simulink model "ff_model"  (R2021a)
settings: Solver=VariableStepAuto  StartTime=0.0  StopTime=data.sim.time  RelTol=1e-7  AbsTol=1e-8
values from neighbouring files (symbols this model uses):
  A_i = [A_sc(1); A_sc(2); A_sc(3); A_sc(1); A_sc(2); A_sc(3);            A_sa; A_sa; A_sa; A_sa]'    [data_setup.m]
  n_i = [eye(3), -eye(3), n_sa, -n_sa, n_sa, -n_sa]    [data_setup.m]
  rhoD = ones(1,10)*0.1    [data_setup.m]
  rhoS = [ones(1,6)*0.5, ones(1,4)*0.8]    [data_setup.m]
undefined symbols (not defined in the file or in its folder): data, F107_avg, F107_day, jdate, km, Kp, omega, s
libraries: sharedutil x10, dspmathops x5, aerolibutil x4, dspmtrx3 x3, aerolibcelestial x2, aerolibatmos2 x2, simulink x1, simulink_extras x1
settings Model: Creator=Francesco  LastModifiedBy=Francesco
settings SolverCC: AutoScaleAbsTol=off
settings DataIOCC: SaveFormat=Array  SaveOutput=off  DSMLogging=off  ReturnWorkspaceOutputsName=simout

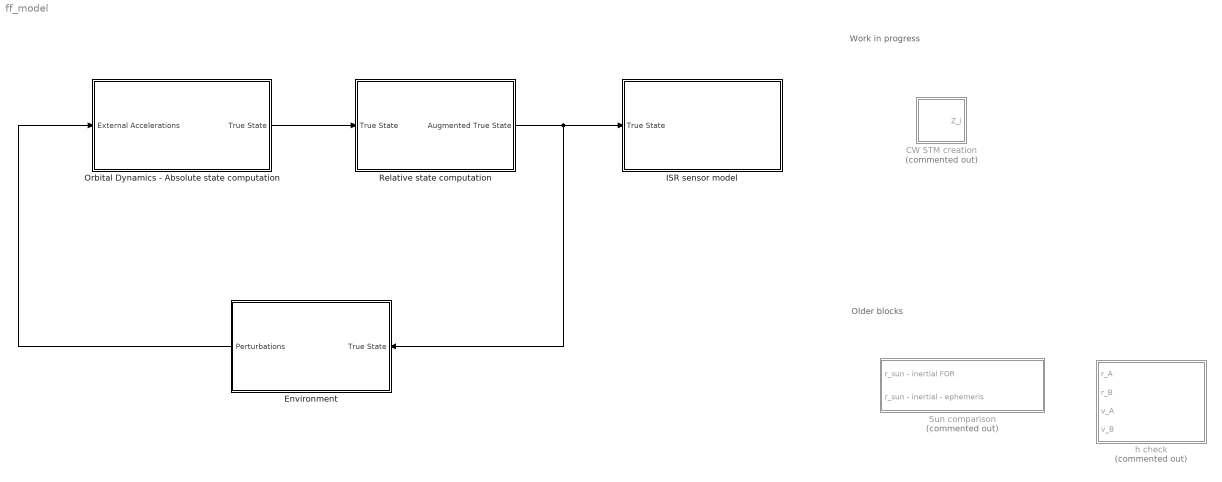
== system ff_model ==
  note: Older blocks
  note: Work in progress
  CW STM creation : Subsystem  Commented=on
  Environment : Subsystem
  ISR sensor model : Subsystem
  "Orbital Dynamics - Absolute state computation " : Subsystem
  Relative state computation : Subsystem
  "Sun comparison " : Subsystem  Commented=on
  h check : Subsystem  Commented=on
  wires:
  Environment/1(Perturbations) -> "Orbital Dynamics - Absolute state computation "/1(External Accelerations)
  "Orbital Dynamics - Absolute state computation "/1(True State) -> Relative state computation/1(True State)
  Relative state computation/1(Augmented True State) -> Environment/1(True State), ISR sensor model/1(True State)

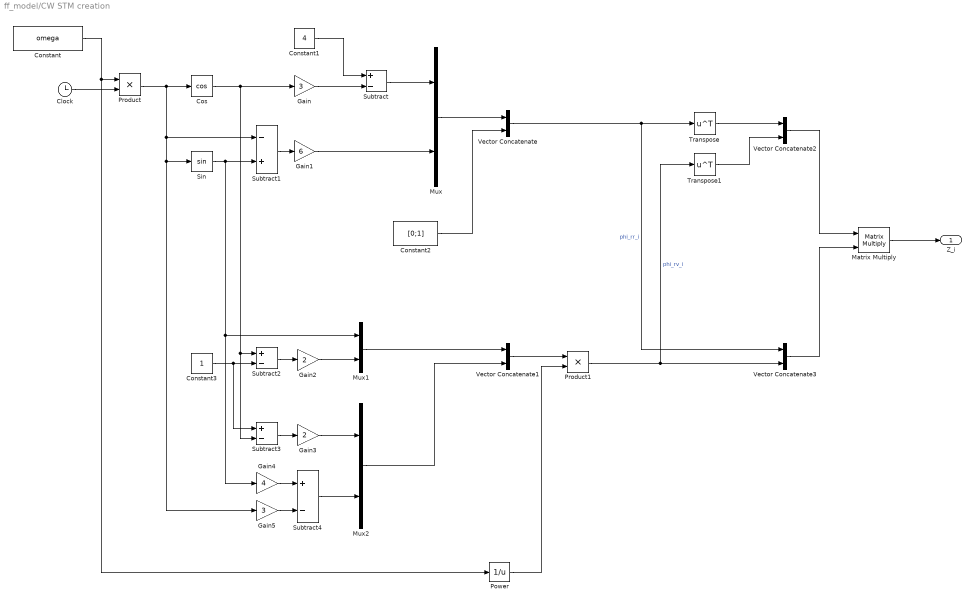
== system ff_model/CW STM creation ==
  Clock : Clock
  Constant : Constant  Value=omega
  Constant1 : Constant  Value=4
  Constant2 : Constant  Value=[0;1]
  Constant3 : Constant
  Cos : Trigonometry  Operator=cos
  Gain : Gain  Gain=3
  Gain1 : Gain  Gain=6
  Gain2 : Gain  Gain=2
  Gain3 : Gain  Gain=2
  Gain4 : Gain  Gain=4
  Gain5 : Gain  Gain=3
  Matrix Multiply : Product  Multiplication=Matrix(*)
  Mux : Mux  Inputs=2
  Mux1 : Mux  Inputs=2
  Mux2 : Mux  Inputs=2
  Power : Math  Operator=reciprocal  SaturateOnIntegerOverflow=on
  Product : Product
  Product1 : Product
  Sin : Trigonometry
  Subtract{,2..4} (4 alike) : Sum  Inputs=+-
  Subtract1 : Sum  Inputs=-+
  Transpose : Math  Operator=transpose  SaturateOnIntegerOverflow=on
  Transpose1 : Math  Operator=transpose  SaturateOnIntegerOverflow=on
  Vector Concatenate : Concatenate  Mode=Multidimensional array  ConcatenateDimension=2
  Vector Concatenate1 : Concatenate  Mode=Multidimensional array  ConcatenateDimension=2
  Vector Concatenate2 : Concatenate  Mode=Multidimensional array
  Vector Concatenate3 : Concatenate  Mode=Multidimensional array  ConcatenateDimension=2
  Z_i : Outport
  wires:
  Product/1 -> Gain5/1, Sin/1, Subtract1/1, Cos/1
  Constant/1 -> Power/1, Product/1
  Gain/1 -> Subtract/2
  Clock/1 -> Product/2
  Subtract/1 -> Mux/1
  Constant2/1 -> Vector Concatenate/2
  Constant1/1 -> Subtract/1
  Cos/1 -> Subtract2/1, Subtract3/2, Gain/1
  Sin/1 -> Gain4/1, Mux1/1, Subtract1/2
  Subtract1/1 -> Gain1/1
  Gain1/1 -> Mux/2
  Mux/1 -> Vector Concatenate/1
  Vector Concatenate/1 -> Vector Concatenate3/1, Transpose/1  "phi_rr_i"
  Constant3/1 -> Subtract3/1, Subtract2/2
  Subtract2/1 -> Gain2/1
  Mux1/1 -> Vector Concatenate1/1
  Gain2/1 -> Mux1/2
  Subtract3/1 -> Gain3/1
  Gain4/1 -> Subtract4/1
  Gain5/1 -> Subtract4/2
  Gain3/1 -> Mux2/1
  Subtract4/1 -> Mux2/2
  Mux2/1 -> Vector Concatenate1/2
  Vector Concatenate1/1 -> Product1/1
  Power/1 -> Product1/2
  Product1/1 -> Transpose1/1, Vector Concatenate3/2  "phi_rv_i"
  Transpose/1 -> Vector Concatenate2/1
  Transpose1/1 -> Vector Concatenate2/2
  Vector Concatenate2/1 -> Matrix Multiply/1
  Vector Concatenate3/1 -> Matrix Multiply/2
  Matrix Multiply/1 -> Z_i/1

== system ff_model/Environment ==
  True State : Inport
  3rd : Scope
  3rd Body : Subsystem
  Drag : Subsystem
  Gain : Gain  Gain=1e-3
  SRP : Subsystem
  Subsystem1 : Subsystem
  Subsystem2 : Subsystem
  Subsystem3 : Subsystem
  Sum : Sum  Inputs=+++
  drag : Scope
  srp : Scope
  Perturbations : Outport
  wires:
  True State/1 -> SRP/1(True State), Drag/1(True State), 3rd Body/1(True State)
  Sum/1 -> Gain/1
  Drag/1(a_drag) -> Subsystem1/1(In1), Sum/3
  3rd Body/1(a_3rd) -> Subsystem2/1(In1), Sum/2
  SRP/1(a_srp) -> Subsystem3/1(In1), Sum/1
  Subsystem3/1(Out1) -> srp/1
  Subsystem2/1(Out1) -> 3rd/1
  Subsystem1/1(Out1) -> drag/1
  Gain/1 -> Perturbations/1

== system ff_model/ISR sensor model ==
  True State : Inport
  Bus Selector : BusSelector  OutputSignals=rel_true_state.posR
  Dot Product : DotProduct  InputSameDT=on  OutDataTypeStr=Inherit: Inherit via internal rule
  Random Number : RandomNumber  Variance=data.sens.sig^2  Seed=354  SampleTime=data.sens.st
  Sqrt : Sqrt  SaturateOnIntegerOverflow=on
  Sum : Sum  Inputs=|++
  To Workspace : ToWorkspace  VariableName=r_meas  SampleTime=-1
      settings: Save2DSignal=2-D array (concatenate along first dimension)
  wires:
  Dot Product/1 -> Sqrt/1
  Sqrt/1 -> Sum/1
  Sum/1 -> To Workspace/1
  Random Number/1 -> Sum/2
  True State/1 -> Bus Selector/1
  Bus Selector/1 -> Dot Product/2, Dot Product/1  "<posR>"

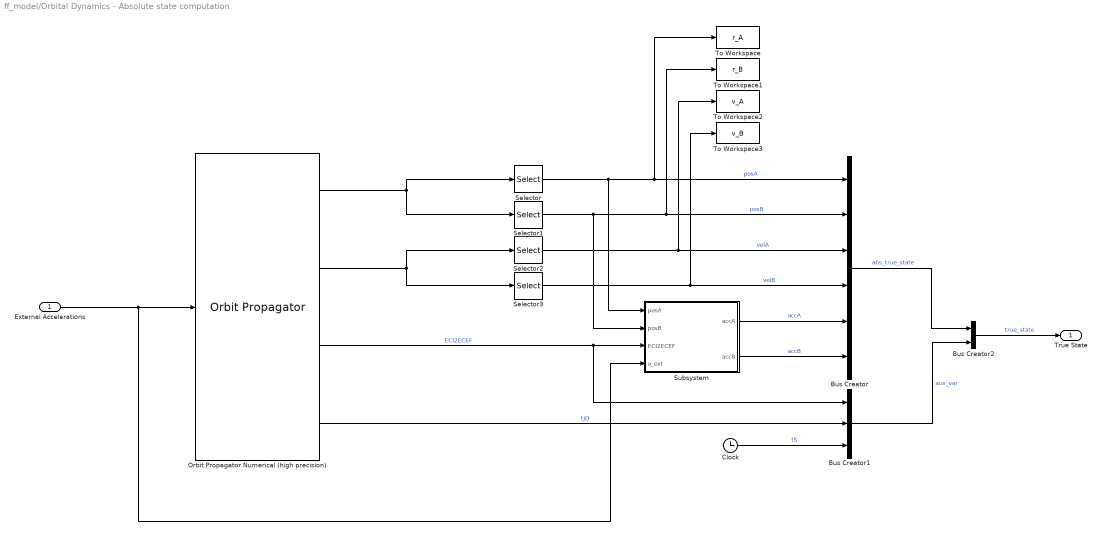
== system ff_model/Orbital Dynamics - Absolute state computation  ==
  External Accelerations : Inport
  Bus Creator : BusCreator  Inputs=6
  Bus Creator1 : BusCreator  Inputs=3
  Bus Creator2 : BusCreator  Inputs=2
  Clock : Clock
  Orbit Propagator Numerical (high precision) : OrbitPropagator  propagator=Numerical (high precision)  accelIn=on  startDate=data.sim.jdate  semiMajorAxis=[data.satA.orbit.a, data.satB.orbit.a]  eccentricity=[data.satA.orbit.e, data.satB.orbit.e]  inclination=[data.satA.orbit.i, data.satB.orbit.i]  raan=[data.satA.orbit.RAAN, data.satB.orbit.RAAN]  argPeriapsis=[data.satA.orbit.om, data.satB.orbit.om]  trueAnomaly=[data.satA.orbit.th, data.satB.orbit.th]  customMu=4.305e13  customJ2=1.0826269e-03  outputTransform=on  units=Metric (km/s)
  Selector : Selector  NumberOfDimensions=2  InputPortWidth=3  IndexOptions=Index vector (dialog),Select all  Indices=1,1  OutputSizes=1,1
  Selector1 : Selector  NumberOfDimensions=2  InputPortWidth=3  IndexOptions=Index vector (dialog),Select all  Indices=2,1  OutputSizes=1,1
  Selector2 : Selector  NumberOfDimensions=2  InputPortWidth=3  IndexOptions=Index vector (dialog),Select all  Indices=1,1  OutputSizes=1,1
  Selector3 : Selector  NumberOfDimensions=2  InputPortWidth=3  IndexOptions=Index vector (dialog),Select all  Indices=2,1  OutputSizes=1,1
  Subsystem : Subsystem
  To Workspace : ToWorkspace  VariableName=r_A  SampleTime=-1
      settings: Save2DSignal=2-D array (concatenate along first dimension)
  To Workspace1 : ToWorkspace  VariableName=r_B  SampleTime=-1
      settings: Save2DSignal=2-D array (concatenate along first dimension)
  To Workspace2 : ToWorkspace  VariableName=v_A  SampleTime=-1
      settings: Save2DSignal=2-D array (concatenate along first dimension)
  To Workspace3 : ToWorkspace  VariableName=v_B  SampleTime=-1
      settings: Save2DSignal=2-D array (concatenate along first dimension)
  True State : Outport
  wires:
  Orbit Propagator Numerical (high precision)/4 -> Bus Creator1/2  "tJD"
  External Accelerations/1 -> Subsystem/4(a_ext), Orbit Propagator Numerical (high precision)/1
  Selector1/1 -> To Workspace1/1, Bus Creator/2, Subsystem/2(posB)  "posB"
  Selector/1 -> To Workspace/1, Bus Creator/1, Subsystem/1(posA)  "posA"
  Orbit Propagator Numerical (high precision)/1 -> Selector/1, Selector1/1
  Orbit Propagator Numerical (high precision)/2 -> Selector2/1, Selector3/1
  Selector2/1 -> To Workspace2/1, Bus Creator/3  "velA"
  Selector3/1 -> To Workspace3/1, Bus Creator/4  "velB"
  Orbit Propagator Numerical (high precision)/3 -> Subsystem/3(ECI2ECEF), Bus Creator1/1  "ECI2ECEF"
  Subsystem/1(accA) -> Bus Creator/5  "accA"
  Subsystem/2(accB) -> Bus Creator/6  "accB"
  Clock/1 -> Bus Creator1/3  "tS"
  Bus Creator1/1 -> Bus Creator2/2  "aux_var"
  Bus Creator/1 -> Bus Creator2/1  "abs_true_state"
  Bus Creator2/1 -> True State/1  "true_state"

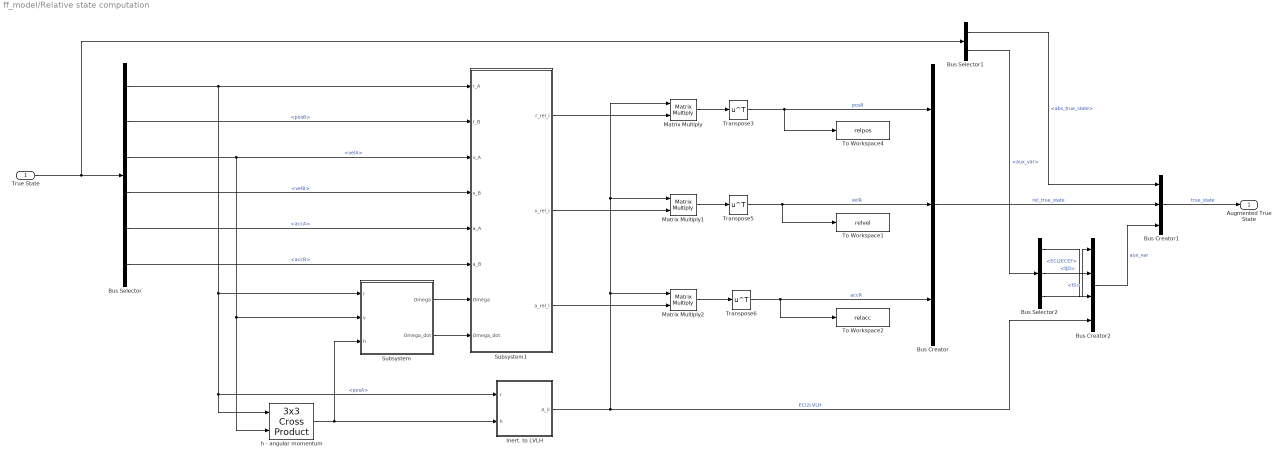
== system ff_model/Relative state computation ==
  True State : Inport
  Bus Creator : BusCreator  Inputs=3
  Bus Creator1 : BusCreator  Inputs=3
  Bus Creator2 : BusCreator  Inputs=4
  Bus Selector : BusSelector  OutputSignals=abs_true_state.posA,abs_true_state.posB,abs_true_state.velA,abs_true_state.velB,abs_true_state.accA,abs_true_state.accB
  Bus Selector1 : BusSelector  OutputSignals=abs_true_state,aux_var
  Bus Selector2 : BusSelector  OutputSignals=ECI2ECEF,tJD,tS
  Inert. to LVLH : Subsystem
  Matrix Multiply : Product  Multiplication=Matrix(*)
  Matrix Multiply1 : Product  Multiplication=Matrix(*)
  Matrix Multiply2 : Product  Multiplication=Matrix(*)
  Subsystem : Subsystem
  Subsystem1 : Subsystem
  To Workspace1 : ToWorkspace  VariableName=relvel  SampleTime=-1
      settings: Save2DSignal=2-D array (concatenate along first dimension)
  To Workspace2 : ToWorkspace  VariableName=relacc  SampleTime=-1
      settings: Save2DSignal=2-D array (concatenate along first dimension)
  To Workspace4 : ToWorkspace  VariableName=relpos  SampleTime=-1
      settings: Save2DSignal=2-D array (concatenate along first dimension)
  Transpose3 : Math  Operator=transpose  SaturateOnIntegerOverflow=on
  Transpose5 : Math  Operator=transpose  SaturateOnIntegerOverflow=on
  Transpose6 : Math  Operator=transpose  SaturateOnIntegerOverflow=on
  h - angular momentum : sharedutil/3x3 Cross Product  aMode=aMode
      settings: SourceProductBaseCode=AE,PW,DR,MT,UV,VE
  Augmented True State : Outport
  wires:
  Inert. to LVLH/1(A_il) -> Bus Creator2/4, Matrix Multiply/1, Matrix Multiply1/1, Matrix Multiply2/1  "ECI2LVLH"
  True State/1 -> Bus Selector1/1, Bus Selector/1
  Bus Selector/4 -> Subsystem1/4(v_B)  "<velB>"
  Bus Selector/5 -> Subsystem1/5(a_A)  "<accA>"
  Bus Selector/2 -> Subsystem1/2(r_B)  "<posB>"
  Bus Selector/1 -> h - angular momentum/1, Inert. to LVLH/1(r), Subsystem/1(r), Subsystem1/1(r_A)  "<posA>"
  Bus Selector/3 -> Subsystem1/3(v_A), h - angular momentum/2, Subsystem/2(v)  "<velA>"
  Bus Selector/6 -> Subsystem1/6(a_B)  "<accB>"
  Subsystem1/3(a_rel_i) -> Matrix Multiply2/2
  Subsystem1/2(v_rel_i) -> Matrix Multiply1/2
  Subsystem1/1(r_rel_i) -> Matrix Multiply/2
  Subsystem/2(Omega_dot) -> Subsystem1/8(Omega_dot)
  Subsystem/1(Omega) -> Subsystem1/7(Omega)
  Matrix Multiply2/1 -> Transpose6/1
  Transpose6/1 -> Bus Creator/3, To Workspace2/1  "accR"
  Transpose3/1 -> To Workspace4/1, Bus Creator/1  "posR"
  Transpose5/1 -> Bus Creator/2, To Workspace1/1  "velR"
  Matrix Multiply1/1 -> Transpose5/1
  Matrix Multiply/1 -> Transpose3/1
  h - angular momentum/1 -> Inert. to LVLH/2(h), Subsystem/3(h)
  Bus Creator/1 -> Bus Creator1/2  "rel_true_state"
  Bus Creator1/1 -> Augmented True State/1  "true_state"
  Bus Selector1/1 -> Bus Creator1/1  "<abs_true_state>"
  Bus Selector1/2 -> Bus Selector2/1  "<aux_var>"
  Bus Selector2/3 -> Bus Creator2/1  "<tS>"
  Bus Selector2/2 -> Bus Creator2/2  "<tJD>"
  Bus Selector2/1 -> Bus Creator2/3  "<ECI2ECEF>"
  Bus Creator2/1 -> Bus Creator1/3  "aux_var"

== system ff_model/Sun comparison  ==
  r_sun - inertial FOR : Inport
  r_sun - inertial - ephemeris : Inport  Port=2
  Acos : Trigonometry  Operator=acos
  Dot Product : DotProduct  InputSameDT=on  OutDataTypeStr=Inherit: Inherit via internal rule
  Radians to Degrees : simulink_extras/Transformations/Radians to Degrees
  Scope : Scope  NumInputPorts=2
  Scope2 : Scope
  wires:
  Acos/1 -> Radians to Degrees/1
  Dot Product/1 -> Acos/1
  r_sun - inertial - ephemeris/1 -> Scope/2, Dot Product/2
  Radians to Degrees/1 -> Scope2/1
  r_sun - inertial FOR/1 -> Scope/1, Dot Product/1

== system ff_model/h check ==
  r_A : Inport
  r_B : Inport  Port=2
  v_A : Inport  Port=3
  v_B : Inport  Port=4
  3x3 Cross Product : sharedutil/3x3 Cross Product  aMode=aMode
      settings: SourceProductBaseCode=AE,PW,DR,MT,UV,VE
  3x3 Cross Product1 : sharedutil/3x3 Cross Product  aMode=aMode
      settings: SourceProductBaseCode=AE,PW,DR,MT,UV,VE
  Scope6 : Scope  Commented=on  NumInputPorts=2
  Subsystem : Subsystem
  Subsystem1 : Subsystem
  wires:
  r_B/1 -> 3x3 Cross Product1/1
  3x3 Cross Product/1 -> Subsystem/1(vec)
  3x3 Cross Product1/1 -> Subsystem1/1(vec)
  Subsystem1/1(norm) -> Scope6/2
  Subsystem/1(norm) -> Scope6/1
  v_B/1 -> 3x3 Cross Product1/2
  v_A/1 -> 3x3 Cross Product/2
  r_A/1 -> 3x3 Cross Product/1

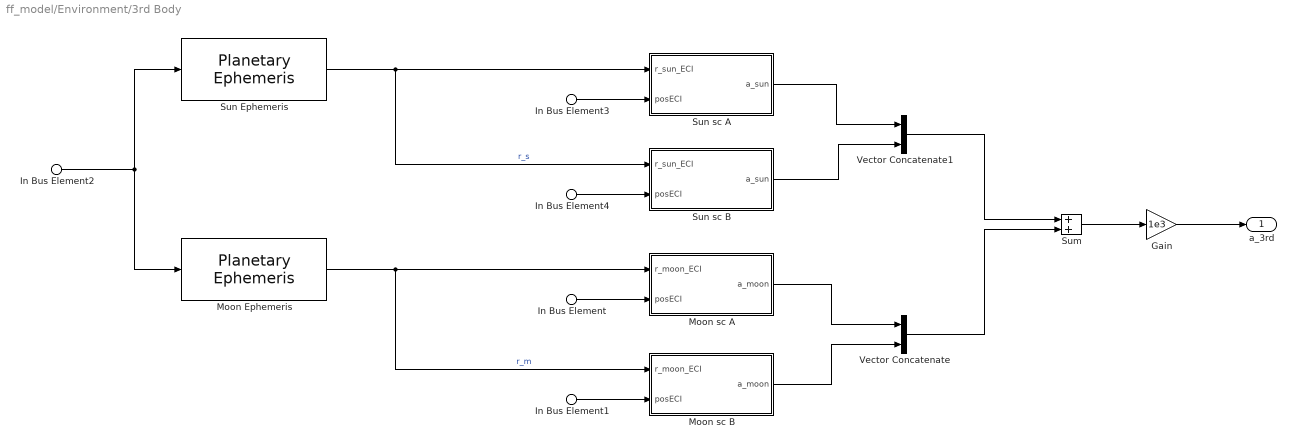
== system ff_model/Environment/3rd Body ==
  In Bus Element : Inport  PortName=True State  Element=abs_true_state.posA
  In Bus Element3 : Inport  PortName=True State  Element=abs_true_state.posA
  In Bus Element1 : Inport  PortName=True State  Element=abs_true_state.posB
  In Bus Element4 : Inport  PortName=True State  Element=abs_true_state.posB
  In Bus Element2 : Inport  PortName=True State  Element=aux_var.tJD
  Gain : Gain  Gain=1e3
  Moon Ephemeris : aerolibcelestial/Planetary Ephemeris  kmflag=km,km/s  epochflag=Julian date  de=DE405  nCenter=Earth  nTarget=Moon  errorflag=Error  velflag=off
      settings: SourceProductBaseCode=AE
  "Moon sc A " : Subsystem
  Moon sc B : Subsystem
  Sum : Sum
  Sun Ephemeris : aerolibcelestial/Planetary Ephemeris  kmflag=km,km/s  epochflag=Julian date  de=DE405  nCenter=Earth  nTarget=Sun  errorflag=Error  velflag=off
      settings: SourceProductBaseCode=AE
  Sun sc A : Subsystem
  Sun sc B : Subsystem
  Vector Concatenate : Concatenate  Mode=Multidimensional array
  Vector Concatenate1 : Concatenate  Mode=Multidimensional array
  a_3rd : Outport
  wires:
  In Bus Element2/1 -> Moon Ephemeris/1, Sun Ephemeris/1
  Moon Ephemeris/1 -> Moon sc B/1(r_moon_ECI), "Moon sc A "/1(r_moon_ECI)  "r_m"
  In Bus Element/1 -> "Moon sc A "/2(posECI)
  In Bus Element1/1 -> Moon sc B/2(posECI)
  Vector Concatenate/1 -> Sum/2
  "Moon sc A "/1(a_moon) -> Vector Concatenate/1
  Moon sc B/1(a_moon) -> Vector Concatenate/2
  Sun sc B/1(a_sun) -> Vector Concatenate1/2
  In Bus Element3/1 -> Sun sc A/2(posECI)
  Sun sc A/1(a_sun) -> Vector Concatenate1/1
  Sun Ephemeris/1 -> Sun sc B/1(r_sun_ECI), Sun sc A/1(r_sun_ECI)  "r_s"
  Vector Concatenate1/1 -> Sum/1
  In Bus Element4/1 -> Sun sc B/2(posECI)
  Sum/1 -> Gain/1
  Gain/1 -> a_3rd/1

== system ff_model/Environment/Drag ==
  In Bus Element : Inport  PortName=True State  Element=abs_true_state.posA
  In Bus Element1 : Inport  PortName=True State  Element=abs_true_state.posB
  In Bus Element2 : Inport  PortName=True State  Element=abs_true_state.velA
  In Bus Element3 : Inport  PortName=True State  Element=abs_true_state.velB
  In Bus Element4 : Inport  PortName=True State  Element=aux_var.ECI2ECEF
  Density sc A : Subsystem
  Density sc B : Subsystem
  Drag sc A : Subsystem
  Drag sc B : Subsystem
  Vector Concatenate : Concatenate  Mode=Multidimensional array
  check rho Jacchia : Subsystem  Commented=on
  rho comp : Scope  Commented=on  NumInputPorts=2
  a_drag : Outport
  wires:
  In Bus Element1/1 -> Drag sc B/3(posECI), Density sc B/2(posECI)
  In Bus Element4/1 -> Density sc A/1(ECI2ECEF), Density sc B/1(ECI2ECEF)
  In Bus Element/1 -> Drag sc A/3(posECI), check rho Jacchia/2(vec), Density sc A/2(posECI)
  Drag sc A/1(a_drag) -> Vector Concatenate/1
  Drag sc B/1(a_drag) -> Vector Concatenate/2
  Vector Concatenate/1 -> a_drag/1
  Density sc B/1(rho) -> Drag sc B/2(rho)
  Density sc A/1(rho) -> check rho Jacchia/1(In1), Drag sc A/2(rho)
  In Bus Element2/1 -> Drag sc A/1(velECI)
  In Bus Element3/1 -> Drag sc B/1(velECI)
  check rho Jacchia/1(Out1) -> rho comp/1
  check rho Jacchia/2(Out2) -> rho comp/2

== system ff_model/Environment/SRP ==
  True State : Inport
  Bus Selector : BusSelector  OutputSignals=aux_var.ECI2LVLH,abs_true_state.posA
  SRP : Subsystem
  Sun Position : Subsystem
  Transpose : Math  Operator=transpose  SaturateOnIntegerOverflow=on
  Vector Concatenate : Concatenate  Mode=Multidimensional array
  a_srp : Outport
  wires:
  Vector Concatenate/1 -> a_srp/1
  True State/1 -> Bus Selector/1
  Sun Position/1(r_sun - inertial FOR) -> SRP/2(r_sun - inertial FOR)
  Transpose/1 -> Vector Concatenate/2, Vector Concatenate/1
  SRP/1(a_SRP_Inert) -> Transpose/1
  Sun Position/2(Shadow) -> SRP/3(Shadow)
  Bus Selector/2 -> Sun Position/1(r_sc - inert FOR)  "<posA>"
  Bus Selector/1 -> SRP/1(A_il)  "<ECI2LVLH>"

== system ff_model/Environment/Subsystem1 ==
  In1 : Inport
  Extract Diagonal : dspmtrx3/Extract Diagonal
      settings: SourceProductBaseCode=DS
  Matrix Multiply : Product  Multiplication=Matrix(*)
  Sqrt : Sqrt  SaturateOnIntegerOverflow=on
  Transpose : Math  Operator=transpose  SaturateOnIntegerOverflow=on
  Out1 : Outport
  wires:
  In1/1 -> Transpose/1, Matrix Multiply/1
  Transpose/1 -> Matrix Multiply/2
  Matrix Multiply/1 -> Extract Diagonal/1
  Extract Diagonal/1 -> Sqrt/1
  Sqrt/1 -> Out1/1

== system ff_model/Environment/Subsystem2 ==
  In1 : Inport
  Extract Diagonal : dspmtrx3/Extract Diagonal
      settings: SourceProductBaseCode=DS
  Matrix Multiply : Product  Multiplication=Matrix(*)
  Sqrt : Sqrt  SaturateOnIntegerOverflow=on
  Transpose : Math  Operator=transpose  SaturateOnIntegerOverflow=on
  Out1 : Outport
  wires:
  In1/1 -> Transpose/1, Matrix Multiply/1
  Transpose/1 -> Matrix Multiply/2
  Matrix Multiply/1 -> Extract Diagonal/1
  Extract Diagonal/1 -> Sqrt/1
  Sqrt/1 -> Out1/1

== system ff_model/Environment/Subsystem3 ==
  In1 : Inport
  Extract Diagonal : dspmtrx3/Extract Diagonal
      settings: SourceProductBaseCode=DS
  Matrix Multiply : Product  Multiplication=Matrix(*)
  Sqrt : Sqrt  SaturateOnIntegerOverflow=on
  Transpose : Math  Operator=transpose  SaturateOnIntegerOverflow=on
  Out1 : Outport
  wires:
  In1/1 -> Transpose/1, Matrix Multiply/1
  Transpose/1 -> Matrix Multiply/2
  Matrix Multiply/1 -> Extract Diagonal/1
  Extract Diagonal/1 -> Sqrt/1
  Sqrt/1 -> Out1/1

== system ff_model/Orbital Dynamics - Absolute state computation /Subsystem ==
  posA : Inport
  posB : Inport  Port=2
  ECI2ECEF : Inport  Port=3
  a_ext : Inport  Port=4
  Gain : Gain  Gain=1e3
  Quaternion Rotation : aerolibutil/Quaternion Rotation
  Quaternion Rotation1 : aerolibutil/Quaternion Rotation
  Selector : Selector  NumberOfDimensions=2  InputPortWidth=3  IndexOptions=Index vector (dialog),Select all  Indices=1,1  OutputSizes=1,1
  Selector1 : Selector  NumberOfDimensions=2  InputPortWidth=3  IndexOptions=Index vector (dialog),Select all  Indices=2,1  OutputSizes=1,1
  Spherical Harmonic Gravity Model : SHGravity
  Sum : Sum  Inputs=|++
  Transpose : Math  Operator=transpose  SaturateOnIntegerOverflow=on
  Vector Concatenate : Concatenate  Mode=Multidimensional array  ConcatenateDimension=2
  accA : Outport
  accB : Outport  Port=2
  wires:
  Quaternion Rotation/1 -> Vector Concatenate/1
  Spherical Harmonic Gravity Model/1 -> Sum/1
  ECI2ECEF/1 -> Quaternion Rotation1/1, Quaternion Rotation/1
  posA/1 -> Quaternion Rotation/2
  posB/1 -> Quaternion Rotation1/2
  Vector Concatenate/1 -> Transpose/1
  Quaternion Rotation1/1 -> Vector Concatenate/2
  Transpose/1 -> Gain/1
  a_ext/1 -> Sum/2
  Sum/1 -> Selector1/1, Selector/1
  Selector/1 -> accA/1  "accA"
  Selector1/1 -> accB/1  "accB"
  Gain/1 -> Spherical Harmonic Gravity Model/1

== system ff_model/Relative state computation/Inert. to LVLH ==
  r : Inport
  h : Inport  Port=2
  3x3 Cross Product1 : sharedutil/3x3 Cross Product  aMode=aMode
      settings: SourceProductBaseCode=AE,PW,DR,MT,UV,VE
  Normalization : dspmathops/Normalization  NormType=2-norm  Bias=1e-10  NormOver=Each row  Dimension=1  roundingMode=Floor  overflowMode=off  accumDataTypeStr=Inherit: Same as product output  accumLastDataTypeStr=Inherit: Same as product output  outputDataTypeStr=Inherit: Same as product output  outputMin=[]  outputMax=[]  outputLastDataTypeStr=Inherit: Same as product output
  Normalization2 : dspmathops/Normalization  NormType=2-norm  Bias=1e-10  NormOver=Each row  Dimension=1  roundingMode=Floor  overflowMode=off  accumDataTypeStr=Inherit: Same as product output  accumLastDataTypeStr=Inherit: Same as product output  outputDataTypeStr=Inherit: Same as product output  outputMin=[]  outputMax=[]  outputLastDataTypeStr=Inherit: Same as product output
  Transpose : Math  Operator=transpose  SaturateOnIntegerOverflow=on
  Transpose1 : Math  Operator=transpose  SaturateOnIntegerOverflow=on
  Vector Concatenate : Concatenate  NumInputs=3  Mode=Multidimensional array
  A_il : Outport
  wires:
  Normalization2/1 -> 3x3 Cross Product1/1, Transpose/1
  h/1 -> Normalization2/1
  3x3 Cross Product1/1 -> Transpose1/1
  Normalization/1 -> Vector Concatenate/1, 3x3 Cross Product1/2  "x_hat"
  Vector Concatenate/1 -> A_il/1
  r/1 -> Normalization/1
  Transpose1/1 -> Vector Concatenate/2  "y_hat"
  Transpose/1 -> Vector Concatenate/3  "z_hat"

== system ff_model/Relative state computation/Subsystem ==
  r : Inport
  v : Inport  Port=2
  h : Inport  Port=3
  Divide : Product  Inputs=*/
  Divide1 : Product  Inputs=*/
  Dot Product : DotProduct  InputSameDT=on  OutDataTypeStr=Inherit: Inherit via internal rule
  Dot Product1 : DotProduct  InputSameDT=on  OutDataTypeStr=Inherit: Inherit via internal rule
  Gain2 : Gain  Gain=-2
  Product : Product
  Omega : Outport
  Omega_dot : Outport  Port=2
  wires:
  Product/1 -> Omega_dot/1  "Omega_dot"
  Divide1/1 -> Product/2  "Omega"
  Dot Product1/1 -> Gain2/1
  r/1 -> Dot Product/2, Dot Product1/2, Dot Product/1
  h/1 -> Divide/1
  v/1 -> Dot Product1/1
  Gain2/1 -> Divide1/1
  Divide/1 -> Product/1, Omega/1  "Omega"
  Dot Product/1 -> Divide1/2, Divide/2

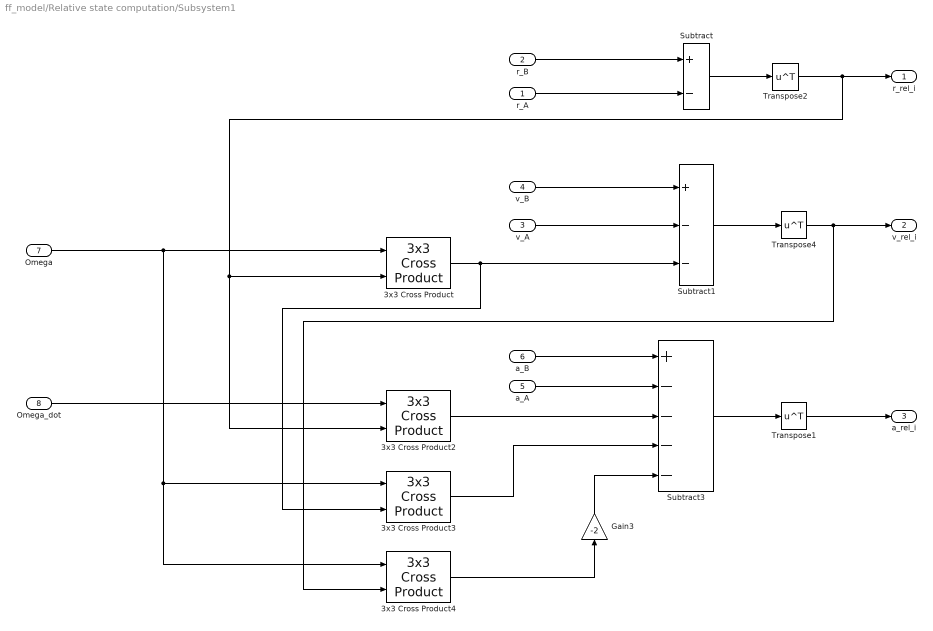
== system ff_model/Relative state computation/Subsystem1 ==
  r_A : Inport
  r_B : Inport  Port=2
  v_A : Inport  Port=3
  v_B : Inport  Port=4
  a_A : Inport  Port=5
  a_B : Inport  Port=6
  Omega : Inport  Port=7
  Omega_dot : Inport  Port=8
  3x3 Cross Product{,2..4} (4 alike) : sharedutil/3x3 Cross Product  aMode=aMode
      settings: SourceProductBaseCode=AE,PW,DR,MT,UV,VE
  Gain3 : Gain  Gain=-2
  Subtract : Sum  Inputs=+-
  Subtract1 : Sum  Inputs=+--
  Subtract3 : Sum  Inputs=+----
  Transpose1 : Math  Operator=transpose  SaturateOnIntegerOverflow=on
  Transpose2 : Math  Operator=transpose  SaturateOnIntegerOverflow=on
  Transpose4 : Math  Operator=transpose  SaturateOnIntegerOverflow=on
  r_rel_i : Outport
  v_rel_i : Outport  Port=2
  a_rel_i : Outport  Port=3
  wires:
  Omega/1 -> 3x3 Cross Product4/1, 3x3 Cross Product3/1, 3x3 Cross Product/1
  Subtract1/1 -> Transpose4/1
  Subtract/1 -> Transpose2/1
  Transpose2/1 -> 3x3 Cross Product/2, 3x3 Cross Product2/2, r_rel_i/1
  3x3 Cross Product/1 -> Subtract1/3, 3x3 Cross Product3/2
  Transpose4/1 -> 3x3 Cross Product4/2, v_rel_i/1
  r_B/1 -> Subtract/1
  Gain3/1 -> Subtract3/5
  3x3 Cross Product2/1 -> Subtract3/3
  3x3 Cross Product4/1 -> Gain3/1
  3x3 Cross Product3/1 -> Subtract3/4
  r_A/1 -> Subtract/2
  v_A/1 -> Subtract1/2
  Omega_dot/1 -> 3x3 Cross Product2/1
  a_A/1 -> Subtract3/2
  a_B/1 -> Subtract3/1
  v_B/1 -> Subtract1/1
  Subtract3/1 -> Transpose1/1
  Transpose1/1 -> a_rel_i/1

== system ff_model/h check/Subsystem ==
  vec : Inport
  Dot Product : DotProduct  InputSameDT=on  OutDataTypeStr=Inherit: Inherit via internal rule
  Sqrt : Sqrt  SaturateOnIntegerOverflow=on
  norm : Outport
  wires:
  Dot Product/1 -> Sqrt/1
  vec/1 -> Dot Product/2, Dot Product/1
  Sqrt/1 -> norm/1

== system ff_model/h check/Subsystem1 ==
  vec : Inport
  Dot Product : DotProduct  InputSameDT=on  OutDataTypeStr=Inherit: Inherit via internal rule
  Sqrt : Sqrt  SaturateOnIntegerOverflow=on
  norm : Outport
  wires:
  Dot Product/1 -> Sqrt/1
  vec/1 -> Dot Product/2, Dot Product/1
  Sqrt/1 -> norm/1

== system ff_model/Environment/3rd Body/Moon sc A  ==
  r_moon_ECI : Inport
  posECI : Inport  Port=2
  Constant : Constant  Value=data.env.mi_moon
  Constant1 : Constant  Value=3
  Constant2 : Constant  Value=3
  Divide : Product  Inputs=*/
  Divide1 : Product  Inputs=*/
  Power : Math  Operator=pow  SaturateOnIntegerOverflow=on
  Power1 : Math  Operator=pow  SaturateOnIntegerOverflow=on
  Product : Product
  Subsystem : Subsystem
  Subsystem1 : Subsystem
  Subtract : Sum  Inputs=+-
  Subtract1 : Sum  Inputs=+-
  a_moon : Outport
  wires:
  Divide1/1 -> Subtract1/2
  r_moon_ECI/1 -> Subtract/1, Subsystem1/1(vec), Divide1/1
  Constant1/1 -> Power/2
  Subtract/1 -> Subsystem/1(vec), Divide/1  "r_sc_m"
  Power/1 -> Divide/2
  Divide/1 -> Subtract1/1
  Power1/1 -> Divide1/2
  Constant2/1 -> Power1/2
  Subsystem1/1(norm) -> Power1/1
  Constant/1 -> Product/1
  Subtract1/1 -> Product/2
  Subsystem/1(norm) -> Power/1
  posECI/1 -> Subtract/2
  Product/1 -> a_moon/1

== system ff_model/Environment/3rd Body/Moon sc B ==
  r_moon_ECI : Inport
  posECI : Inport  Port=2
  Constant : Constant  Value=data.env.mi_moon
  Constant1 : Constant  Value=3
  Constant2 : Constant  Value=3
  Divide : Product  Inputs=*/
  Divide1 : Product  Inputs=*/
  Power : Math  Operator=pow  SaturateOnIntegerOverflow=on
  Power1 : Math  Operator=pow  SaturateOnIntegerOverflow=on
  Product : Product
  Subsystem : Subsystem
  Subsystem1 : Subsystem
  Subtract : Sum  Inputs=+-
  Subtract1 : Sum  Inputs=+-
  a_moon : Outport
  wires:
  Divide1/1 -> Subtract1/2
  r_moon_ECI/1 -> Subtract/1, Subsystem1/1(vec), Divide1/1
  Constant1/1 -> Power/2
  Subtract/1 -> Subsystem/1(vec), Divide/1  "r_sc_m"
  Power/1 -> Divide/2
  Divide/1 -> Subtract1/1
  Power1/1 -> Divide1/2
  Constant2/1 -> Power1/2
  Subsystem1/1(norm) -> Power1/1
  Constant/1 -> Product/1
  Subtract1/1 -> Product/2
  Subsystem/1(norm) -> Power/1
  posECI/1 -> Subtract/2
  Product/1 -> a_moon/1

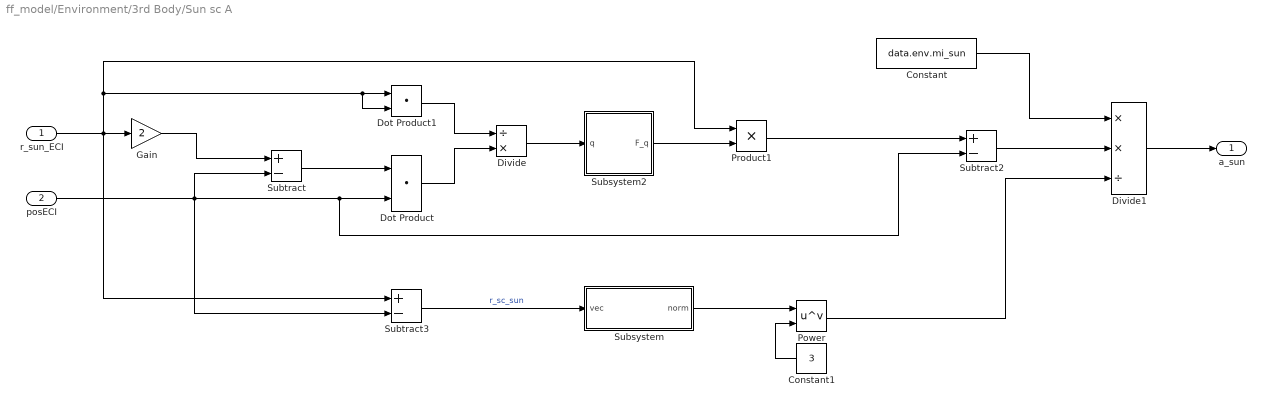
== system ff_model/Environment/3rd Body/Sun sc A ==
  r_sun_ECI : Inport
  posECI : Inport  Port=2
  Constant : Constant  Value=data.env.mi_sun
  Constant1 : Constant  Value=3
  Divide : Product  Inputs=/*
  Divide1 : Product  Inputs=**/
  Dot Product : DotProduct  InputSameDT=on  OutDataTypeStr=Inherit: Inherit via internal rule
  Dot Product1 : DotProduct  InputSameDT=on  OutDataTypeStr=Inherit: Inherit via internal rule
  Gain : Gain  Gain=2
  Power : Math  Operator=pow  SaturateOnIntegerOverflow=on
  Product1 : Product
  Subsystem : Subsystem
  Subsystem2 : Subsystem
  Subtract : Sum  Inputs=+-
  Subtract2 : Sum  Inputs=+-
  Subtract3 : Sum  Inputs=+-
  a_sun : Outport
  wires:
  r_sun_ECI/1 -> Product1/1, Dot Product1/2, Dot Product1/1, Subtract3/1, Gain/1
  Gain/1 -> Subtract/1
  Subtract/1 -> Dot Product/1
  Dot Product1/1 -> Divide/1
  Dot Product/1 -> Divide/2
  Divide/1 -> Subsystem2/1(q)
  Subsystem2/1(F_q) -> Product1/2
  Product1/1 -> Subtract2/1
  posECI/1 -> Subtract3/2, Subtract2/2, Dot Product/2, Subtract/2
  Power/1 -> Divide1/3
  Constant1/1 -> Power/2
  Subtract3/1 -> Subsystem/1(vec)  "r_sc_sun"
  Subsystem/1(norm) -> Power/1
  Constant/1 -> Divide1/1
  Subtract2/1 -> Divide1/2
  Divide1/1 -> a_sun/1

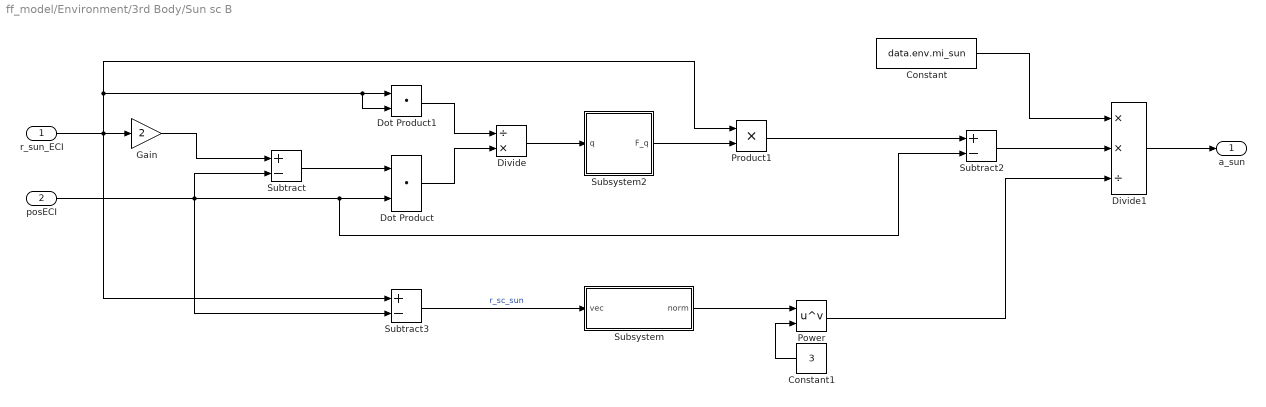
== system ff_model/Environment/3rd Body/Sun sc B ==
  r_sun_ECI : Inport
  posECI : Inport  Port=2
  Constant : Constant  Value=data.env.mi_sun
  Constant1 : Constant  Value=3
  Divide : Product  Inputs=/*
  Divide1 : Product  Inputs=**/
  Dot Product : DotProduct  InputSameDT=on  OutDataTypeStr=Inherit: Inherit via internal rule
  Dot Product1 : DotProduct  InputSameDT=on  OutDataTypeStr=Inherit: Inherit via internal rule
  Gain : Gain  Gain=2
  Power : Math  Operator=pow  SaturateOnIntegerOverflow=on
  Product1 : Product
  Subsystem : Subsystem
  Subsystem2 : Subsystem
  Subtract : Sum  Inputs=+-
  Subtract2 : Sum  Inputs=+-
  Subtract3 : Sum  Inputs=+-
  a_sun : Outport
  wires:
  r_sun_ECI/1 -> Product1/1, Dot Product1/2, Dot Product1/1, Subtract3/1, Gain/1
  Gain/1 -> Subtract/1
  Subtract/1 -> Dot Product/1
  Dot Product1/1 -> Divide/1
  Dot Product/1 -> Divide/2
  Divide/1 -> Subsystem2/1(q)
  Subsystem2/1(F_q) -> Product1/2
  Product1/1 -> Subtract2/1
  posECI/1 -> Subtract3/2, Subtract2/2, Dot Product/2, Subtract/2
  Power/1 -> Divide1/3
  Constant1/1 -> Power/2
  Subtract3/1 -> Subsystem/1(vec)  "r_sc_sun"
  Subsystem/1(norm) -> Power/1
  Constant/1 -> Divide1/1
  Subtract2/1 -> Divide1/2
  Divide1/1 -> a_sun/1

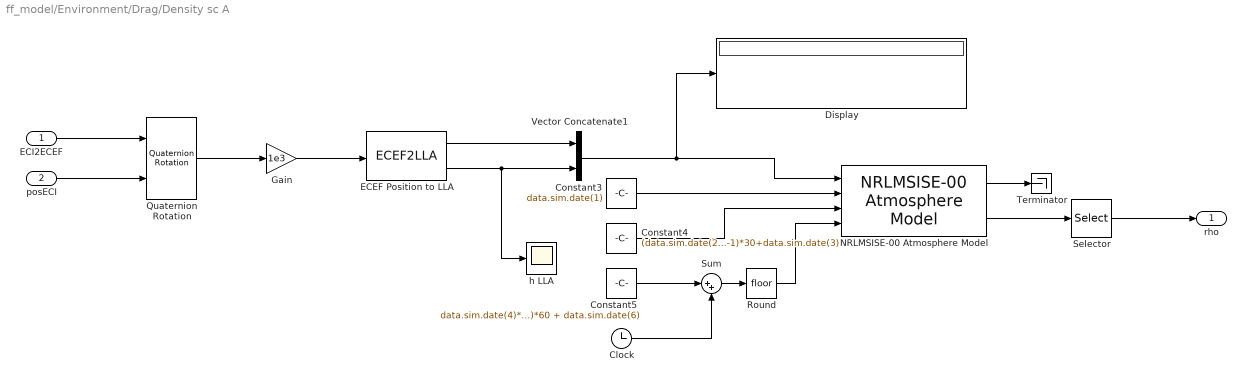
== system ff_model/Environment/Drag/Density sc A ==
  ECI2ECEF : Inport
  posECI : Inport  Port=2
  Clock : Clock
  Constant3 : Constant  Value=data.sim.date(1)
  Constant4 : Constant  Value=(data.sim.date(2)-1)*30+data.sim.date(3)
  Constant5 : Constant  Value=data.sim.date(4)*60*60 + data.sim.date(5)*60 + data.sim.date(6)
  Display : Display
  ECEF Position to LLA : ECEF2LLA
  Gain : Gain  Gain=1e3
  NRLMSISE-00 Atmosphere Model : aerolibatmos2/NRLMSISE-00 Atmosphere Model  units=Metric (MKS)  lst_input=off  flux_ap_input=off  flags_input=Internal  flags=ones(1,23)  oxygen_in=on  action=Warning
      settings: SourceProductBaseCode=AE
  Quaternion Rotation : aerolibutil/Quaternion Rotation
  Round : Rounding
  Selector : Selector  InputPortWidth=9  IndexOptions=Index vector (dialog)  Indices=6  OutputSizes=1
  Sum : Sum  Inputs=|++
  Terminator : Terminator
  Vector Concatenate1 : Concatenate
  h LLA : Scope
  rho : Outport
  wires:
  Constant4/1 -> NRLMSISE-00 Atmosphere Model/3
  Gain/1 -> ECEF Position to LLA/1
  Vector Concatenate1/1 -> Display/1, NRLMSISE-00 Atmosphere Model/1
  Clock/1 -> Sum/2
  NRLMSISE-00 Atmosphere Model/1 -> Terminator/1
  NRLMSISE-00 Atmosphere Model/2 -> Selector/1
  ECEF Position to LLA/1 -> Vector Concatenate1/1
  Constant3/1 -> NRLMSISE-00 Atmosphere Model/2
  Quaternion Rotation/1 -> Gain/1
  Constant5/1 -> Sum/1
  Sum/1 -> Round/1
  ECEF Position to LLA/2 -> h LLA/1, Vector Concatenate1/2
  Selector/1 -> rho/1
  Round/1 -> NRLMSISE-00 Atmosphere Model/4
  posECI/1 -> Quaternion Rotation/2
  ECI2ECEF/1 -> Quaternion Rotation/1

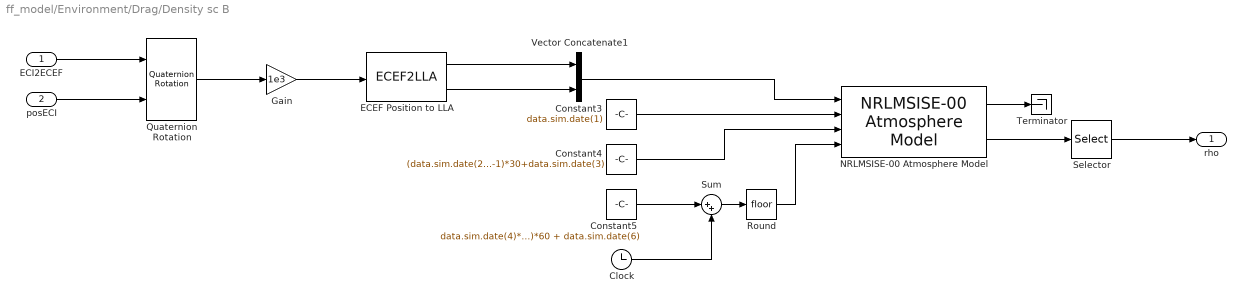
== system ff_model/Environment/Drag/Density sc B ==
  ECI2ECEF : Inport
  posECI : Inport  Port=2
  Clock : Clock
  Constant3 : Constant  Value=data.sim.date(1)
  Constant4 : Constant  Value=(data.sim.date(2)-1)*30+data.sim.date(3)
  Constant5 : Constant  Value=data.sim.date(4)*60*60 + data.sim.date(5)*60 + data.sim.date(6)
  ECEF Position to LLA : ECEF2LLA
  Gain : Gain  Gain=1e3
  NRLMSISE-00 Atmosphere Model : aerolibatmos2/NRLMSISE-00 Atmosphere Model  units=Metric (MKS)  lst_input=off  flux_ap_input=off  flags_input=Internal  flags=ones(1,23)  oxygen_in=on  action=Warning
      settings: SourceProductBaseCode=AE
  Quaternion Rotation : aerolibutil/Quaternion Rotation
  Round : Rounding
  Selector : Selector  InputPortWidth=9  IndexOptions=Index vector (dialog)  Indices=6  OutputSizes=1
  Sum : Sum  Inputs=|++
  Terminator : Terminator
  Vector Concatenate1 : Concatenate
  rho : Outport
  wires:
  Constant4/1 -> NRLMSISE-00 Atmosphere Model/3
  Gain/1 -> ECEF Position to LLA/1
  Vector Concatenate1/1 -> NRLMSISE-00 Atmosphere Model/1
  Clock/1 -> Sum/2
  NRLMSISE-00 Atmosphere Model/1 -> Terminator/1
  NRLMSISE-00 Atmosphere Model/2 -> Selector/1
  ECEF Position to LLA/1 -> Vector Concatenate1/1
  Constant3/1 -> NRLMSISE-00 Atmosphere Model/2
  Quaternion Rotation/1 -> Gain/1
  Constant5/1 -> Sum/1
  Sum/1 -> Round/1
  ECEF Position to LLA/2 -> Vector Concatenate1/2
  Selector/1 -> rho/1
  Round/1 -> NRLMSISE-00 Atmosphere Model/4
  posECI/1 -> Quaternion Rotation/2
  ECI2ECEF/1 -> Quaternion Rotation/1

== system ff_model/Environment/Drag/Drag sc A ==
  velECI : Inport
  rho : Inport  Port=2
  posECI : Inport  Port=3
  3x3 Cross Product : sharedutil/3x3 Cross Product  aMode=aMode
      settings: SourceProductBaseCode=AE,PW,DR,MT,UV,VE
  Constant : Constant  Value=[0 0 data.env.w_e]
  Constant1 : Constant  Value=-0.5
  Constant2 : Constant  Value=data.satA.BC
  Gain : Gain  Gain=1e3
  Product : Product  Inputs=5
  Subsystem : Subsystem
  Subtract : Sum  Inputs=+-
  a_drag : Outport
  wires:
  Constant1/1 -> Product/1
  Subtract/1 -> Gain/1
  posECI/1 -> 3x3 Cross Product/2
  Constant/1 -> 3x3 Cross Product/1
  Gain/1 -> Subsystem/1(vec), Product/5  "vel_rel_air"
  3x3 Cross Product/1 -> Subtract/2
  Subsystem/1(norm) -> Product/3
  Product/1 -> a_drag/1
  Constant2/1 -> Product/4
  velECI/1 -> Subtract/1
  rho/1 -> Product/2

== system ff_model/Environment/Drag/Drag sc B ==
  velECI : Inport
  rho : Inport  Port=2
  posECI : Inport  Port=3
  3x3 Cross Product : sharedutil/3x3 Cross Product  aMode=aMode
      settings: SourceProductBaseCode=AE,PW,DR,MT,UV,VE
  Constant : Constant  Value=[0 0 data.env.w_e]
  Constant1 : Constant  Value=-0.5
  Constant2 : Constant  Value=data.satB.BC
  Gain : Gain  Gain=1e3
  Product : Product  Inputs=5
  Subsystem : Subsystem
  Subtract : Sum  Inputs=+-
  a_drag : Outport
  wires:
  Constant1/1 -> Product/1
  Subtract/1 -> Gain/1
  posECI/1 -> 3x3 Cross Product/2
  Constant/1 -> 3x3 Cross Product/1
  Gain/1 -> Subsystem/1(vec), Product/5  "vel_rel_air"
  3x3 Cross Product/1 -> Subtract/2
  Subsystem/1(norm) -> Product/3
  Product/1 -> a_drag/1
  Constant2/1 -> Product/4
  velECI/1 -> Subtract/1
  rho/1 -> Product/2

== system ff_model/Environment/Drag/check rho Jacchia ==
  In1 : Inport
  vec : Inport  Port=2
  Constant : Constant  Value=data.env.r_e
  Constant6 : Constant  Value=F107_avg
  Constant7 : Constant  Value=F107_day
  Constant8 : Constant  Value=Kp
  Constant9 : Constant  Value=jdate
  Gain : Gain  Gain=1e3
  Log : Math  Operator=log  SaturateOnIntegerOverflow=on
  Log1 : Math  Operator=log  SaturateOnIntegerOverflow=on
  Subsystem : Subsystem
      settings: PortSchema="{\"entries\":[{\"content\":{\"sides\":[{\"content\":{\"connectorIds\":[\"In1\"]},\"type\":\"ConnectorPlacement.EquallySpacedRectSide\",\"uuid\":\"fad14b86-e979-4d0a-a7c2-7763da4a249a\"},{\"content\":{\"connectorIds\":[],\"side\":\"RIGHT\"},\"type\":\"ConnectorPlacement.EquallySpacedRectSide\",\"uuid\":\"989f86c2-e873-44d8-9617-53b07eed6f09\"},{\"content\":{\"connectorIds\":[\"Out1\"],\"side\":\"TOP\"},\"type\":\"ConnectorPlacement.EquallySpacedRectSide\",\"uuid\":\"b56db859-4edb-4bc6-b5ca-32fc0913a58c\"}]},\"type\":\"ConnectorPlacement.EquallySpacedConnector\",\"uuid\":\"cfe7daa7-9618-4947-8749-dc7cde67e806\"}],\"packageUris\":[\"http://schema.mathworks.com/mf0/Connector/R2020b\"],\"version\":\"1.0\"}"
  Subtract : Sum  Inputs=+-
  density calculator 0-2500 km : MATLAB Function  TreatAsAtomicUnit=on
  h spanne : Scope
  Out1 : Outport
  Out2 : Outport  Port=2
  wires:
  Constant6/1 -> density calculator 0-2500 km/3(F107_avg)
  Constant9/1 -> density calculator 0-2500 km/2(jdate)
  Constant8/1 -> density calculator 0-2500 km/5(Kp)
  density calculator 0-2500 km/1(rho) -> Log1/1
  Gain/1 -> h spanne/1, density calculator 0-2500 km/1(h)
  Constant7/1 -> density calculator 0-2500 km/4(F107_act)
  Subtract/1 -> Gain/1
  Subsystem/1(norm) -> Subtract/1
  Log/1 -> Out1/1
  Constant/1 -> Subtract/2
  Log1/1 -> Out2/1
  vec/1 -> Subsystem/1(vec)
  In1/1 -> Log/1

== system ff_model/Environment/SRP/SRP ==
  A_il : Inport
  r_sun - inertial FOR : Inport  Port=2
  Shadow : Inport  Port=3
  Matrix Multiply : Product  Multiplication=Matrix(*)
  Matrix Multiply1 : Product  Multiplication=Matrix(*)
  Product : Product
  Solar Radiation Pressure : Subsystem  TreatAsAtomicUnit=on
  Transpose1 : Math  Operator=transpose  SaturateOnIntegerOverflow=on
  force to acc : Gain  Gain=1/12
  a_SRP_Inert : Outport
  wires:
  Product/1 -> Solar Radiation Pressure/1(r_sun - body)
  Matrix Multiply/1 -> Product/1
  r_sun - inertial FOR/1 -> Matrix Multiply/2
  Shadow/1 -> Product/2
  A_il/1 -> Transpose1/1, Matrix Multiply/1
  Transpose1/1 -> Matrix Multiply1/1  "LVLH to Inert"
  Matrix Multiply1/1 -> force to acc/1
  force to acc/1 -> a_SRP_Inert/1
  Solar Radiation Pressure/1(F_d_SRP) -> Matrix Multiply1/2

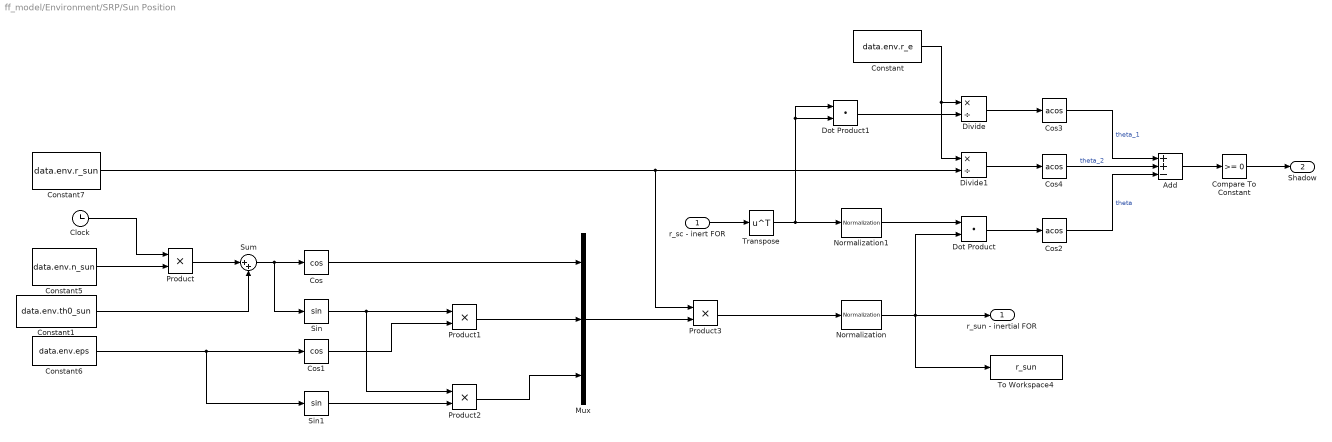
== system ff_model/Environment/SRP/Sun Position ==
  r_sc - inert FOR : Inport
  Add : Sum  Inputs=++-
  Clock : Clock
  Compare To Constant : simulink/Logic and Bit Operations/Compare To Constant  relop=>=  const=0  OutDataTypeStr=boolean
  Constant : Constant  Value=data.env.r_e
  Constant1 : Constant  Value=data.env.th0_sun
  Constant5 : Constant  Value=data.env.n_sun
  Constant6 : Constant  Value=data.env.eps
  Constant7 : Constant  Value=data.env.r_sun
  Cos : Trigonometry  Operator=cos
  Cos1 : Trigonometry  Operator=cos
  Cos2 : Trigonometry  Operator=acos
  Cos3 : Trigonometry  Operator=acos
  Cos4 : Trigonometry  Operator=acos
  Divide : Product  Inputs=*/
  Divide1 : Product  Inputs=*/
  Dot Product : DotProduct  InputSameDT=on  OutDataTypeStr=Inherit: Inherit via internal rule
  Dot Product1 : DotProduct  InputSameDT=on  OutDataTypeStr=Inherit: Inherit via internal rule
  Mux : Mux  Inputs=3
  Normalization : dspmathops/Normalization  NormType=2-norm  Bias=1e-10  NormOver=Each column  Dimension=1  roundingMode=Floor  overflowMode=off  accumDataTypeStr=Inherit: Same as product output  accumLastDataTypeStr=Inherit: Same as product output  outputDataTypeStr=Inherit: Same as product output  outputMin=[]  outputMax=[]  outputLastDataTypeStr=Inherit: Same as product output
  Normalization1 : dspmathops/Normalization  NormType=2-norm  Bias=1e-10  NormOver=Each column  Dimension=1  roundingMode=Floor  overflowMode=off  accumDataTypeStr=Inherit: Same as product output  accumLastDataTypeStr=Inherit: Same as product output  outputDataTypeStr=Inherit: Same as product output  outputMin=[]  outputMax=[]  outputLastDataTypeStr=Inherit: Same as product output
  Product{,1..3} (4 alike) : Product
  Sin : Trigonometry
  Sin1 : Trigonometry
  Sum : Sum  Inputs=|++
  To Workspace4 : ToWorkspace  VariableName=r_sun  SampleTime=-1
      settings: Save2DSignal=2-D array (concatenate along first dimension)
  Transpose : Math  Operator=transpose  SaturateOnIntegerOverflow=on
  r_sun - inertial FOR : Outport  VectorParamsAs1DForOutWhenUnconnected=off
  Shadow : Outport  Port=2  VectorParamsAs1DForOutWhenUnconnected=off
  wires:
  Sin/1 -> Product2/1, Product1/1
  Cos/1 -> Mux/1
  Mux/1 -> Product3/2
  Constant6/1 -> Sin1/1, Cos1/1
  Product2/1 -> Mux/3
  Product1/1 -> Mux/2
  Product3/1 -> Normalization/1
  Constant5/1 -> Product/2
  Cos1/1 -> Product1/2
  Clock/1 -> Product/1
  Sin1/1 -> Product2/2
  Constant7/1 -> Product3/1, Divide1/2
  Normalization/1 -> r_sun - inertial FOR/1, To Workspace4/1, Dot Product/2
  r_sc - inert FOR/1 -> Transpose/1
  Dot Product/1 -> Cos2/1
  Cos2/1 -> Add/3  "theta"
  Constant/1 -> Divide1/1, Divide/1
  Divide/1 -> Cos3/1
  Divide1/1 -> Cos4/1
  Cos3/1 -> Add/1  "theta_1"
  Cos4/1 -> Add/2  "theta_2"
  Add/1 -> Compare To Constant/1
  Compare To Constant/1 -> Shadow/1
  Dot Product1/1 -> Divide/2
  Product/1 -> Sum/1
  Sum/1 -> Sin/1, Cos/1
  Constant1/1 -> Sum/2
  Normalization1/1 -> Dot Product/1
  Transpose/1 -> Normalization1/1, Dot Product1/1, Dot Product1/2

== system ff_model/Environment/3rd Body/Moon sc A /Subsystem ==
  vec : Inport
  Dot Product : DotProduct  InputSameDT=on  OutDataTypeStr=Inherit: Inherit via internal rule
  Sqrt : Sqrt  SaturateOnIntegerOverflow=on
  norm : Outport
  wires:
  vec/1 -> Dot Product/2, Dot Product/1
  Sqrt/1 -> norm/1
  Dot Product/1 -> Sqrt/1

== system ff_model/Environment/3rd Body/Moon sc A /Subsystem1 ==
  vec : Inport
  Dot Product : DotProduct  InputSameDT=on  OutDataTypeStr=Inherit: Inherit via internal rule
  Sqrt : Sqrt  SaturateOnIntegerOverflow=on
  norm : Outport
  wires:
  vec/1 -> Dot Product/2, Dot Product/1
  Sqrt/1 -> norm/1
  Dot Product/1 -> Sqrt/1

== system ff_model/Environment/3rd Body/Moon sc B/Subsystem ==
  vec : Inport
  Dot Product : DotProduct  InputSameDT=on  OutDataTypeStr=Inherit: Inherit via internal rule
  Sqrt : Sqrt  SaturateOnIntegerOverflow=on
  norm : Outport
  wires:
  vec/1 -> Dot Product/2, Dot Product/1
  Sqrt/1 -> norm/1
  Dot Product/1 -> Sqrt/1

== system ff_model/Environment/3rd Body/Moon sc B/Subsystem1 ==
  vec : Inport
  Dot Product : DotProduct  InputSameDT=on  OutDataTypeStr=Inherit: Inherit via internal rule
  Sqrt : Sqrt  SaturateOnIntegerOverflow=on
  norm : Outport
  wires:
  vec/1 -> Dot Product/2, Dot Product/1
  Sqrt/1 -> norm/1
  Dot Product/1 -> Sqrt/1

== system ff_model/Environment/3rd Body/Sun sc A/Subsystem ==
  vec : Inport
  Dot Product : DotProduct  InputSameDT=on  OutDataTypeStr=Inherit: Inherit via internal rule
  Sqrt : Sqrt  SaturateOnIntegerOverflow=on
  norm : Outport
  wires:
  vec/1 -> Dot Product/2, Dot Product/1
  Sqrt/1 -> norm/1
  Dot Product/1 -> Sqrt/1

== system ff_model/Environment/3rd Body/Sun sc A/Subsystem2 ==
  q : Inport
  Constant3 : Constant  Value=3
  Constant4 : Constant
  Constant5 : Constant  Value=3/2
  Divide2 : Product  Inputs=*/*
  Gain : Gain  Gain=3
  Power2 : Math  Operator=pow  SaturateOnIntegerOverflow=on
  Square : Math  Operator=square  SaturateOnIntegerOverflow=on
  Subtract2 : Sum  Inputs=+-+
  Subtract3 : Sum  Inputs=+-
  Sum : Sum
  F_q : Outport
  wires:
  Constant4/1 -> Subtract3/1, Sum/1
  q/1 -> Square/1, Gain/1, Divide2/3, Subtract3/2
  Sum/1 -> Divide2/2
  Gain/1 -> Subtract2/2
  Subtract2/1 -> Divide2/1
  Subtract3/1 -> Power2/1
  Constant3/1 -> Subtract2/3
  Power2/1 -> Sum/2
  Constant5/1 -> Power2/2
  Square/1 -> Subtract2/1
  Divide2/1 -> F_q/1

== system ff_model/Environment/3rd Body/Sun sc B/Subsystem ==
  vec : Inport
  Dot Product : DotProduct  InputSameDT=on  OutDataTypeStr=Inherit: Inherit via internal rule
  Sqrt : Sqrt  SaturateOnIntegerOverflow=on
  norm : Outport
  wires:
  vec/1 -> Dot Product/2, Dot Product/1
  Sqrt/1 -> norm/1
  Dot Product/1 -> Sqrt/1

== system ff_model/Environment/3rd Body/Sun sc B/Subsystem2 ==
  q : Inport
  Constant3 : Constant  Value=3
  Constant4 : Constant
  Constant5 : Constant  Value=3/2
  Divide2 : Product  Inputs=*/*
  Gain : Gain  Gain=3
  Power2 : Math  Operator=pow  SaturateOnIntegerOverflow=on
  Square : Math  Operator=square  SaturateOnIntegerOverflow=on
  Subtract2 : Sum  Inputs=+-+
  Subtract3 : Sum  Inputs=+-
  Sum : Sum
  F_q : Outport
  wires:
  Constant4/1 -> Subtract3/1, Sum/1
  q/1 -> Square/1, Gain/1, Divide2/3, Subtract3/2
  Sum/1 -> Divide2/2
  Gain/1 -> Subtract2/2
  Subtract2/1 -> Divide2/1
  Subtract3/1 -> Power2/1
  Constant3/1 -> Subtract2/3
  Power2/1 -> Sum/2
  Constant5/1 -> Power2/2
  Square/1 -> Subtract2/1
  Divide2/1 -> F_q/1

== system ff_model/Environment/Drag/Drag sc A/Subsystem ==
  vec : Inport
  Dot Product : DotProduct  InputSameDT=on  OutDataTypeStr=Inherit: Inherit via internal rule
  Sqrt : Sqrt  SaturateOnIntegerOverflow=on
  norm : Outport
  wires:
  vec/1 -> Dot Product/2, Dot Product/1
  Sqrt/1 -> norm/1
  Dot Product/1 -> Sqrt/1

== system ff_model/Environment/Drag/Drag sc B/Subsystem ==
  vec : Inport
  Dot Product : DotProduct  InputSameDT=on  OutDataTypeStr=Inherit: Inherit via internal rule
  Sqrt : Sqrt  SaturateOnIntegerOverflow=on
  norm : Outport
  wires:
  vec/1 -> Dot Product/2, Dot Product/1
  Sqrt/1 -> norm/1
  Dot Product/1 -> Sqrt/1

== system ff_model/Environment/Drag/check rho Jacchia/Subsystem ==
  vec : Inport
  Dot Product : DotProduct  InputSameDT=on  OutDataTypeStr=Inherit: Inherit via internal rule
  Sqrt : Sqrt  SaturateOnIntegerOverflow=on
  norm : Outport
  wires:
  vec/1 -> Dot Product/2, Dot Product/1
  Sqrt/1 -> norm/1
  Dot Product/1 -> Sqrt/1

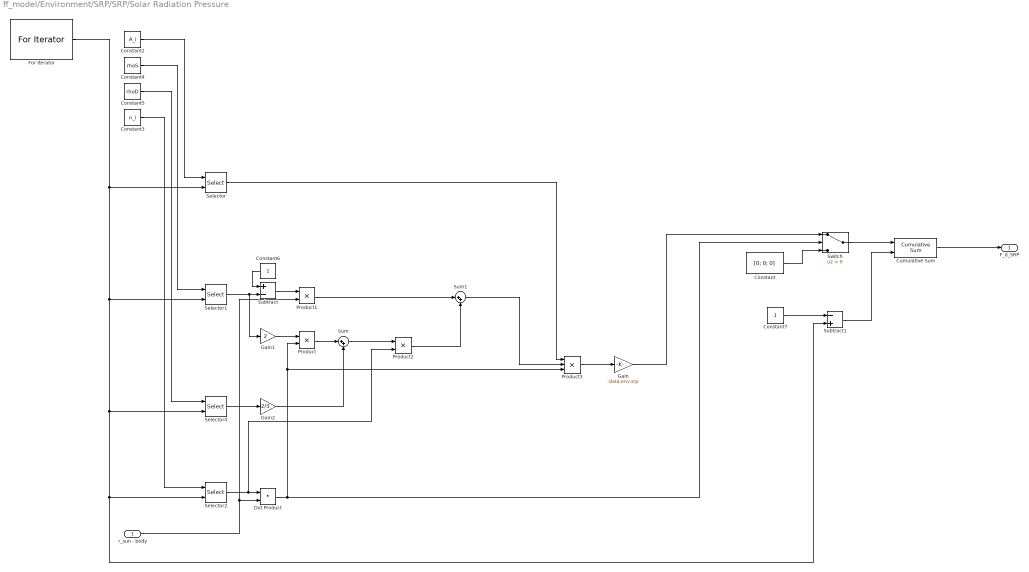
== system ff_model/Environment/SRP/SRP/Solar Radiation Pressure ==
  r_sun - body : Inport
  Constant : Constant  Value=[0; 0; 0]
  Constant2 : Constant  Value=A_i
  Constant3 : Constant  Value=n_i
  Constant4 : Constant  Value=rhoS
  Constant5 : Constant  Value=rhoD
  Constant6 : Constant
  Constant7 : Constant
  Cumulative Sum : dspmathops/Cumulative Sum  dim=Channels (running sum)  reset_popup=Falling edge  roundingMode=Floor  overflowMode=off  outputDataTypeStr=Inherit: Same as accumulator  outputMin=[]  outputMax=[]  outputLastDataTypeStr=Inherit: Same as accumulator
  Dot Product : DotProduct  InputSameDT=on  OutDataTypeStr=Inherit: Inherit via internal rule
  For Iterator : ForIterator  IterationLimit=length(A_i)
  Gain : Gain  Gain=-data.env.srp
  Gain1 : Gain  Gain=2
  Gain2 : Gain  Gain=2/3
  Product : Product
  Product1 : Product
  Product2 : Product
  Product3 : Product  Inputs=3
  Selector{,1..2,4} (4 alike) : Selector  NumberOfDimensions=2  InputPortWidth=3  IndexOptions=Select all,Index vector (port)  Indices=[1 3],1  OutputSizes=1,1
  Subtract : Sum  Inputs=+-
  Subtract1 : Sum  Inputs=-+
  Sum : Sum  Inputs=|++
  Sum1 : Sum  Inputs=|++
  Switch : Switch  Criteria=u2 > Threshold
  F_d_SRP : Outport  VectorParamsAs1DForOutWhenUnconnected=off
  wires:
  For Iterator/1 -> Selector/2, Subtract1/2, Selector2/2, Selector4/2, Selector1/2
  Selector/1 -> Product3/1
  Constant3/1 -> Selector2/1
  Selector2/1 -> Product2/2, Dot Product/1
  Constant2/1 -> Selector/1
  r_sun - body/1 -> Product1/2, Dot Product/2
  Constant4/1 -> Selector1/1
  Constant5/1 -> Selector4/1
  Selector1/1 -> Subtract/2, Gain1/1
  Constant6/1 -> Subtract/1
  Subtract/1 -> Product1/1
  Dot Product/1 -> Product/2, Product3/3, Switch/2
  Gain1/1 -> Product/1
  Selector4/1 -> Gain2/1
  Product/1 -> Sum/1
  Gain2/1 -> Sum/2
  Sum/1 -> Product2/1
  Product1/1 -> Sum1/1
  Product2/1 -> Sum1/2
  Sum1/1 -> Product3/2
  Product3/1 -> Gain/1
  Constant/1 -> Switch/3
  Gain/1 -> Switch/1
  Switch/1 -> Cumulative Sum/1
  Subtract1/1 -> Cumulative Sum/2
  Constant7/1 -> Subtract1/1
  Cumulative Sum/1 -> F_d_SRP/1

== matlab function ff_model/Environment/Drag/check rho Jacchia/density calculator 0-2500 km ==
  data: h input; rho output; jdate input; F107_avg input; F107_act input; Kp input
%This function combinates Jacchia J71 and Exponential Atmosphere for
%calculating density in the band [0;2500] km
%A transition function should be introduced to avoid discontinuities

function rho = unirho(h,jdate,F107_avg,F107_act,Kp)
h=h/1000; %conversion [m] to [km]
rho=0;

%from 0 to 100 km of altitude use Exponential Atmosphere
    if h<100 && h>=0
        rho=expAtm(h);
    end

%from 100 to 2500 km of altitude use Jacchia J71
    if h>=100 && h<=2500
        rho=J71_density_simulink(h,jdate,F107_avg,F107_act,Kp);
    end

%A warning is printed if a negative altitude is predicted by
%the simulation (due to simulink discrete stopping criterion)
    if h<0
        fprintf('Warning: mismatched density, altitude: %3.2e km',h)
        rho=1.225;
    end

end
